simulink model "greenhouse_model"  (R2022a)
settings: Solver=VariableStepAuto  StartTime=0.0  StopTime=3600  RelTol=1e-3
values from neighbouring files (symbols this model uses):
  A = 1000    [ControlSIM.m]    (also in ProjectSim.m; greenhouseEnv.m)
  alpha = 0.125    [ControlSIM.m]    (also in ProjectSim.m; greenhouseEnv.m)
  Cp = 1006    [ControlSIM.m]    (also in ProjectSim.m; greenhouseEnv.m)
  gamma = 2257    [ControlSIM.m]    (also in ProjectSim.m; greenhouseEnv.m)
  Qfog = Qfog_e    (= 18)    [ProjectSim.m]
  Qfog_e = 18    [ProjectSim.m]
  rho = 1.2    [ControlSIM.m]    (also in ProjectSim.m; greenhouseEnv.m)
  Sr = Sr_e    (= 300)    [ProjectSim.m]    (also in StepSimulation.m = [143.6157;215.91;253.55;93.2419]; greenhouseEnv.m = this.State(3))
  Sr_e = 300    [ProjectSim.m]
  Tin_e = Tout_e + (1/(rho*Vt_e*Cp + U*A))*(Si - gamma*Qfog_e)    (= 31.9964933103)    [ProjectSim.m]
  Tout = Tout_e    (= 25)    [ProjectSim.m]
  Tout_e = 25    [ProjectSim.m]
  U = 4    [ControlSIM.m]    (also in ProjectSim.m = 25; greenhouseEnv.m)
  V = 4000    [ControlSIM.m]    (also in ProjectSim.m; greenhouseEnv.m)
  Vt = Vt_e    (= 10)    [ProjectSim.m]
  Vt_e = 10    [ProjectSim.m]
  win_e = Wout_e + (1/Vt_e)*(Qfog_e + E)    (= 7.46149756314)    [ProjectSim.m]
  wout = Wout_e    (= 4)    [ProjectSim.m]
  Wout_e = 4    [ProjectSim.m]
libraries: cstblocks x2
settings Model: Creator=Aaron  LastModifiedBy=Aaron

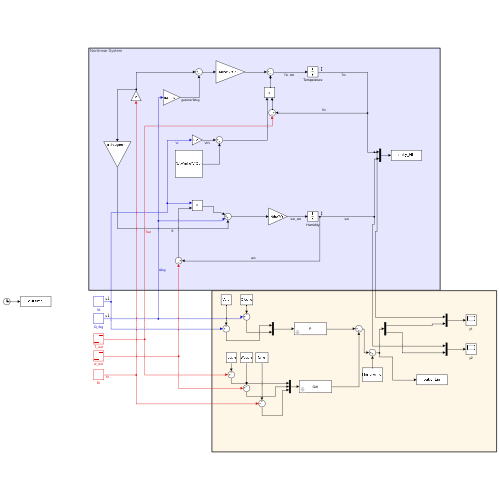
[thumbnail: Simulink's stored preview of the top-level diagram]
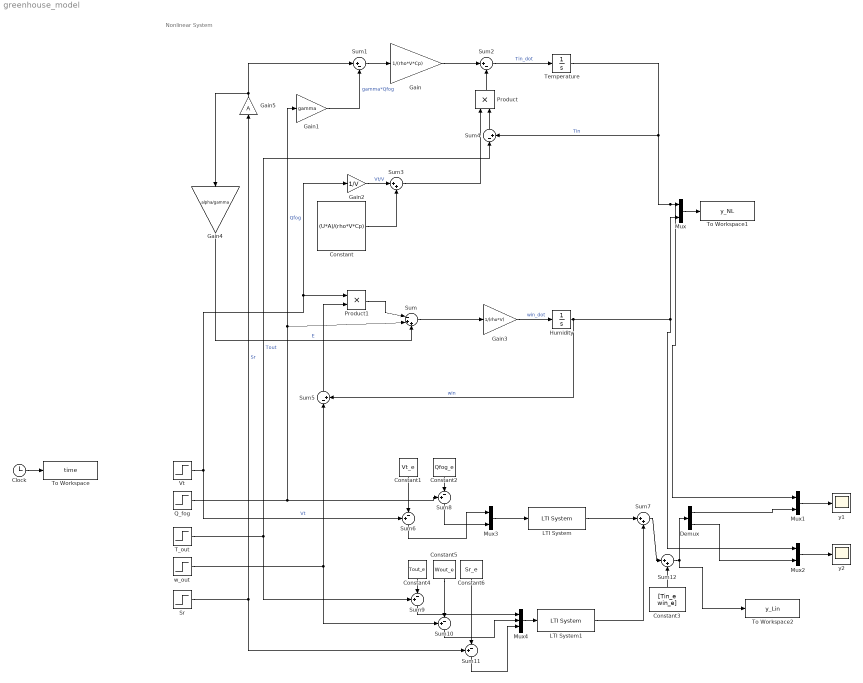
== system greenhouse_model ==
  note: Nonlinear System
  Clock : Clock
  Constant : Constant  Value=(U*A)/(rho*V*Cp)
  Constant1 : Constant  Value=Vt_e
  Constant2 : Constant  Value=Qfog_e
  Constant3 : Constant  Value=[Tin_e win_e]
  Constant4 : Constant  Value=Tout_e
  Constant5 : Constant  Value=Wout_e
  Constant6 : Constant  Value=Sr_e
  Demux : Demux  Outputs=2
  Gain : Gain  Gain=1/(rho*V*Cp)
  Gain1 : Gain  Gain=gamma
  Gain2 : Gain  Gain=1/V
  Gain3 : Gain  Gain=1/(rho*V)
  Gain4 : Gain  Gain=alpha/gamma
  Gain5 : Gain  Gain=A
  Humidity : Integrator  InitialCondition=win_e
  LTI System : cstblocks/LTI System  sys=P  IC=[]
  LTI System1 : cstblocks/LTI System  sys=Gdt  IC=[]
  Mux{,1..3} (4 alike) : Mux  Inputs=2
  Mux4 : Mux  Inputs=3
  Product : Product
  Product1 : Product
  Q_fog : Step  Time=0  After=Qfog  SampleTime=0
  Sr : Step  Time=0  After=Sr  SampleTime=0
  Sum : Sum  Inputs=|-++
  Sum1 : Sum  Inputs=|+-
  Sum{6,8..11} (5 alike) : Sum  Inputs=+-|
  Sum12 : Sum  Inputs=|++
  Sum2 : Sum  Inputs=|+-
  Sum3 : Sum  Inputs=|++
  Sum4 : Sum  Inputs=|-+
  Sum5 : Sum  Inputs=|-+
  Sum7 : Sum  Inputs=|++
  T_out : Step  Time=0  After=Tout  SampleTime=0
  Temperature : Integrator  InitialCondition=Tin_e
  To Workspace : ToWorkspace  VariableName=time  SaveFormat=Timeseries  SampleTime=-1
  To Workspace1 : ToWorkspace  VariableName=y_NL  SaveFormat=Timeseries  SampleTime=-1
  To Workspace2 : ToWorkspace  VariableName=y_Lin  SaveFormat=Timeseries  SampleTime=-1
  Vt : Step  Time=0  After=Vt-4  SampleTime=0
  w_out : Step  Time=0  After=wout  SampleTime=0
  y1 : Scope
  y2 : Scope
  wires:
  Q_fog/1 -> Gain1/1, Sum/2, Sum8/1  "Qfog"
  Gain1/1 -> Sum1/2  "gamma*Qfog"
  Sum1/1 -> Gain/1
  Sum2/1 -> Temperature/1  "Tin_dot"
  Gain/1 -> Sum2/1
  Temperature/1 -> Mux1/1, Mux/1, Sum4/2  "Tin"
  Vt/1 -> Sum6/1, Gain2/1, Product1/1  "Vt"
  Gain2/1 -> Sum3/1  "Vt/V"
  Constant/1 -> Sum3/2
  Product/1 -> Sum2/2
  Sum3/1 -> Product/1
  Sum4/1 -> Product/2
  T_out/1 -> Sum9/1, Sum4/1  "Tout"
  Sum/1 -> Gain3/1
  Gain3/1 -> Humidity/1  "win_dot"
  Humidity/1 -> Sum5/2, Mux2/1, Mux/2  "win"
  Gain4/1 -> Sum/3  "E"
  w_out/1 -> Sum5/1, Sum10/1
  Sum5/1 -> Product1/2
  Product1/1 -> Sum/1
  Clock/1 -> To Workspace/1
  Sr/1 -> Sum11/1, Gain5/1  "Sr"
  Gain5/1 -> Gain4/1, Sum1/1
  Mux/1 -> To Workspace1/1
  Mux1/1 -> y1/1
  Mux2/1 -> y2/1
  Constant1/1 -> Sum6/2
  Constant2/1 -> Sum8/2
  Mux3/1 -> LTI System/1
  Sum8/1 -> Mux3/2
  Sum6/1 -> Mux3/1
  Demux/2 -> Mux2/2
  LTI System/1 -> Sum7/1
  Demux/1 -> Mux1/2
  Constant4/1 -> Sum9/2
  Constant5/1 -> Sum10/2
  Constant6/1 -> Sum11/2
  Mux4/1 -> LTI System1/1
  Sum9/1 -> Mux4/1
  Sum10/1 -> Mux4/2
  Sum11/1 -> Mux4/3
  LTI System1/1 -> Sum7/2
  Sum12/1 -> To Workspace2/1, Demux/1
  Sum7/1 -> Sum12/1
  Constant3/1 -> Sum12/2
